simulink model "seminarskimpup"  (R2020b)
settings: Solver=VariableStepAuto  StartTime=0.0  StopTime=.5  RelTol=1e-3
undefined symbols (not defined in the file or in its folder): DiscIntNeverNeededParam
libraries: simulink x1
settings Model: Creator=Toni  LastModifiedBy=Toni

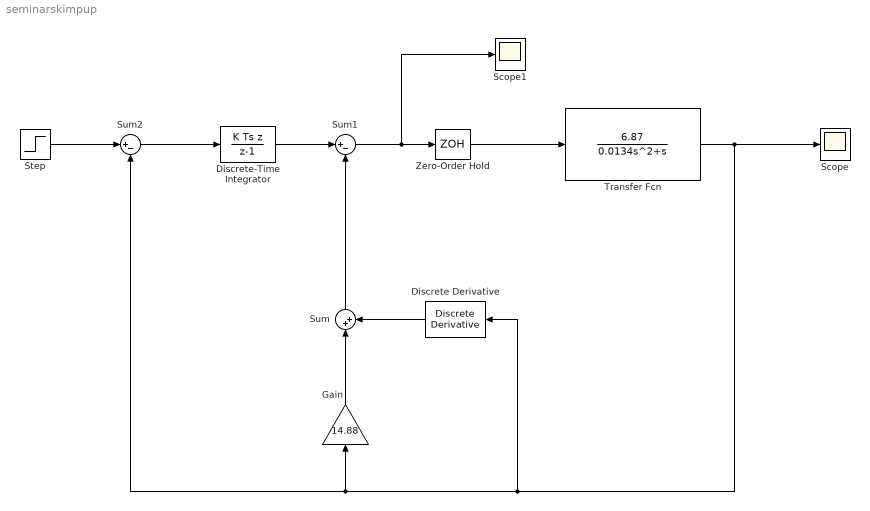
== system seminarskimpup ==
  Discrete Derivative : simulink/Discrete/Discrete Derivative  gainval=0.14136  ICPrevScaledInput=0.0  OutMin=[]  OutMax=[]  OutDataType=fixdt(1, 16)  OutScaling=2^-10  DoSatur=off
  Discrete-Time Integrator : DiscreteIntegrator  IntegratorMethod=Integration: Backward Euler  gainval=270.5454  SampleTime=-1  ICPrevOutput=DiscIntNeverNeededParam  ICPrevScaledInput=DiscIntNeverNeededParam
  Gain : Gain  Gain=14.88
  Scope : Scope
  Scope1 : Scope
  Step : Step  Time=0.005  SampleTime=0
  Sum : Sum  Inputs=|++
  Sum1 : Sum  Inputs=|+-
  Sum2 : Sum  Inputs=|+-
  Transfer Fcn : TransferFcn  Numerator=[6.87]  Denominator=[0.0134 1 0]
  Zero-Order Hold : ZeroOrderHold  SampleTime=0.005
  wires:
  Sum/1 -> Sum1/2
  Discrete Derivative/1 -> Sum/2
  Discrete-Time Integrator/1 -> Sum1/1
  Sum2/1 -> Discrete-Time Integrator/1
  Gain/1 -> Sum/1
  Transfer Fcn/1 -> Scope/1, Discrete Derivative/1, Sum2/2, Gain/1
  Sum1/1 -> Scope1/1, Zero-Order Hold/1
  Zero-Order Hold/1 -> Transfer Fcn/1
  Step/1 -> Sum2/1
